simulink library "THBMemory"  (R2018b)
settings: Solver=ode45  StartTime=0.0  StopTime=10.0  RelTol=1e-3  EnableMultiTasking=on
settings Model: Creator=lena.frank  LastModifiedBy=P41573
settings DataIOCC: LimitDataPoints=on  SaveFormat=Array  SignalLoggingSaveFormat=ModelDataLogs
settings OptimizationCC: ExpressionDepthLimit=2147483647  LifeSpan=inf
settings DebuggingCC: UnderspecifiedInitializationDetection=Classic  MergeDetectMultiDrivingBlocksExec=none  SolverPrmCheckMsg=warning  FcnCallInpInsideContextMsg=warning  StateNameClashWarn=warning  SFUnexpectedBacktrackingDiag=warning  SFNoUnconditionalDefaultTransitionDiag=warning  SFExecutionAtInitializationDiag=none
settings HardwareCC: ProdBitPerPointer=32  ProdBitPerSizeT=32  ProdBitPerPtrDiffT=32  ProdLargestAtomicFloat=None  ProdIntDivRoundTo=Undefined  ProdEndianess=Unspecified  ProdWordSize=32  ProdHWDeviceType=32-bit Generic
settings ModelReferenceCC: PropagateSignalLabelsOutOfModel=off
settings SFSimCC: SimUseLocalCustomCode=off
settings RTWCC: RTWUseLocalCustomCode=off
settings CodeAppCC: StateflowObjectComments=on
settings GRTTargetCC: TargetLangStandard=C89/C90 (ANSI)  GeneratePreprocessorConditionals=Disable all  CombineOutputUpdateFcns=off  GRTInterface=on
settings ConfigComp: CovMetricSettings=dw  CovHtmlReporting=on  CovSaveCumulativeToWorkspaceVar=on  CovSaveSingleToWorkspaceVar=on  CovExternalEMLEnable=off

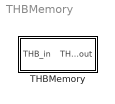
== system THBMemory ==
  THBMemory : Subsystem  InitFcn=load('THB.mat');  mask(THB Memory){ID=20001, T=20, mdot=0, p=1e5, FluidType=1, FluidMix=0, d=0.01, c=0, l=0, q=0, LH=1000, H=0, Annotation_ID=off, Annotation_T=off, Annotation_mdot=off, Annotation_p=off, Annotation_FluidType=off, Annotation_FluidMix=off, Annotation_d=off, Annotation_c=off, Annotation_l=off, Annotation_q=off, Annotation_LH=off, Annotation_H=off}
      mask prompts: ID "Fluid ID [1]"; T "Temperature [°C]"; mdot "Mass flow rate [kg/s]"; p "Pressure [Pa]"; FluidType "Fluid type [enum]"; FluidMix "Fluid mix [1]"; d "Diameter of the last piece [m]"; c "Constant pressure drop coefficient [Pa]"; l "Linear pressure drop coefficient [Pa/(kg/s)]"; q "Quadratic pressure drop coefficient [Pa/(kg/s)²]"; LH "Hydraulic inductance [1/m]"; H "Geodetic height [m]"; Annotation_ID "Fluid ID as annotation"; Annotation_T "Temperature as annoation"; Annotation_mdot "Mass flow rate as annoation"; Annotation_p "Pressure as annotation"; Annotation_FluidType "Fluid type as annotation"; Annotation_FluidMix "Fluid mix as annotation"; Annotation_d "Diameter of the last piece as annotation"; Annotation_c "Constant pressure drop coefficient as annotation"; Annotation_l "Linear pressure drop coefficient as annotation"; Annotation_q "Quadratic pressure drop coefficient as annotation"; Annotation_LH "Hydraulic inductance as annotation"; Annotation_H "Geodetic height as annotation"
      mask help: This is a memory block for a complete THB.
      mask init:
      | %annotations    
      | MaskValues=get_param(gcb,'MaskValues');
      | AnnotationString='';
      | if strcmp(MaskValues{13},'on') %ID
      |     if ~isempty(AnnotationString)
      |         AnnotationString=[AnnotationString,sprintf('\n')];
      |     end
      |     AnnotationString=[AnnotationString,'ID ',MaskValues{1}];
      | end
      |     
      | if strcmp(MaskValues{14},'on') %T
      |     if ~isempty(AnnotationString)
      |         AnnotationString=[AnnotationString,sprintf('\n')];
      |     end
      |     AnnotationString=[AnnotationString,MaskValues{2}, ' °C temperature'];
      | end
      |     
      | if strcmp(MaskValues{15},'on') %T
      |     if ~isempty(AnnotationString)
      |         AnnotationString=[AnnotationString,sprintf('\n')];
      |     end
      |     AnnotationString=[AnnotationString,MaskValues{3}, ' kg/s mass flow rate'];
      | end
      |     
      | if strcmp(MaskValues{16},'on') %p
      |     if ~isempty(AnnotationString)
      |         AnnotationString=[AnnotationString,sprintf('\n')];
      |     end
      |     AnnotationString=[AnnotationString,MaskValues{4}, ' Pa pressure'];
      | end
      | 
      | if strcmp(MaskValues{17},'on') %type
      |     if ~isempty(AnnotationString)
      |         AnnotationString=[AnnotationString,sprintf('\n')];
      |     end
      |     AnnotationString=[AnnotationString,'fluid type ',MaskValues{5}];
      | end
      |     
      | if strcmp(MaskValues{18},'on') %mix
      |     if ~isempty(AnnotationString)
      |         AnnotationString=[AnnotationString,sprintf('\n')];
      |     end
      |     AnnotationString=[AnnotationString,MaskValues{6}, ' fluid mix'];
      | end
      |     
      | if strcmp(MaskValues{19},'on') %d
      |     if ~isempty(AnnotationString)
      |         AnnotationString=[AnnotationString,sprintf('\n')];
      |     end
      |     AnnotationString=[AnnotationString,MaskValues{7}, ' m diameter last piece'];
      | end
      |     
      | if strcmp(MaskValues{20},'on') %c
      |     if ~isempty(AnnotationString)
      |         AnnotationString=[AnnotationString,sprintf('\n')];
      |     end
      |     AnnotationString=[AnnotationString,MaskValues{8}, ' Pa constant pressure loss coefficient'];
      | end
      |     
      | if strcmp(MaskValues{21},'on') %l
      |     if ~isempty(AnnotationString)
      |         AnnotationString=[AnnotationString,sprintf('\n')];
      |     end
      |     AnnotationString=[AnnotationString,MaskValues{9}, ' Pa/(kg/s) linear pressure loss coefficient'];
      | end
      |     
      | if strcmp(MaskValues{22},'on') %q
      |     if ~isempty(AnnotationString)
      |         AnnotationString=[AnnotationString,sprintf('\n')];
      |     end
      |     AnnotationString=[AnnotationString,MaskValues{10}, ' Pa/(kg/s)² quadratic pressure loss coefficient'];
      | end
      |     
      | if strcmp(MaskValues{23},'on') %LH
      |     if ~isempty(AnnotationString)
      |         AnnotationString=[AnnotationString,sprintf('\n')];
      |     end
      |     AnnotationString=[AnnotationString,MaskValues{11}, ' 1/m hydraulic inductance'];
      | end
      |     
      | if strcmp(MaskValues{24},'on') %H
      |     if ~isempty(AnnotationString)
      |         AnnotationString=[AnnotationString,sprintf('\n')];
      |     end
      |     AnnotationString=[AnnotationString,MaskValues{12}, ' m geodetic height'];
      | end
      |     
      | set_param(gcb,'AttributesFormatString',AnnotationString);
      | 
      | clear MaskValues AnnotationString;
      mask Help: web(fullfile(path_carnot('help'),'THBMemory.html'),'-helpbrowser')
      mask DialogControl ParameterTabVar0 Prompt: values
      mask DialogControl ParameterTabVar01 Prompt: annotations

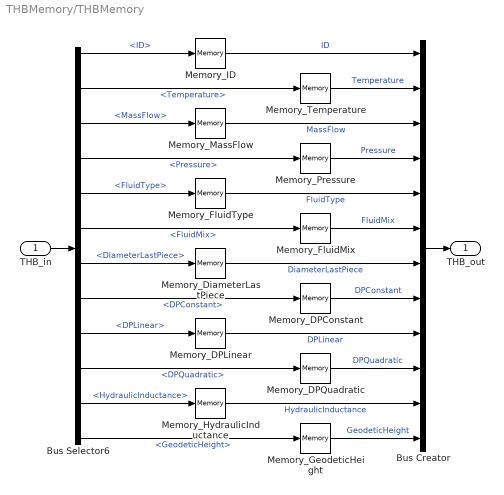
== system THBMemory/THBMemory ==
  THB_in : Inport  OutDataTypeStr=Bus: THB
  Bus Creator : BusCreator  Inputs=12
  Bus Selector6 : BusSelector  OutputSignals=ID,Temperature,MassFlow,Pressure,FluidType,FluidMix,DiameterLastPiece,DPConstant,DPLinear,DPQuadratic,HydraulicInductance,GeodeticHeight
  Memory_DPConstant : Memory  InitialCondition=c
  Memory_DPLinear : Memory  InitialCondition=l
  Memory_DPQuadratic : Memory  InitialCondition=q
  Memory_DiameterLastPiece : Memory  InitialCondition=d
  Memory_FluidMix : Memory  InitialCondition=FluidMix
  Memory_FluidType : Memory  InitialCondition=FluidType
  Memory_GeodeticHeight : Memory  InitialCondition=H
  Memory_HydraulicInductance : Memory  InitialCondition=LH
  Memory_ID : Memory  InitialCondition=ID
  Memory_MassFlow : Memory  InitialCondition=mdot
  Memory_Pressure : Memory  InitialCondition=p
  Memory_Temperature : Memory  InitialCondition=T
  THB_out : Outport
  wires:
  THB_in/1 -> Bus Selector6/1
  Bus Creator/1 -> THB_out/1
  Memory_HydraulicInductance/1 -> Bus Creator/11  "HydraulicInductance"
  Bus Selector6/11 -> Memory_HydraulicInductance/1  "<HydraulicInductance>"
  Memory_DPQuadratic/1 -> Bus Creator/10  "DPQuadratic"
  Bus Selector6/10 -> Memory_DPQuadratic/1  "<DPQuadratic>"
  Memory_DPLinear/1 -> Bus Creator/9  "DPLinear"
  Bus Selector6/9 -> Memory_DPLinear/1  "<DPLinear>"
  Memory_DPConstant/1 -> Bus Creator/8  "DPConstant"
  Bus Selector6/8 -> Memory_DPConstant/1  "<DPConstant>"
  Memory_DiameterLastPiece/1 -> Bus Creator/7  "DiameterLastPiece"
  Bus Selector6/7 -> Memory_DiameterLastPiece/1  "<DiameterLastPiece>"
  Memory_FluidMix/1 -> Bus Creator/6  "FluidMix"
  Bus Selector6/6 -> Memory_FluidMix/1  "<FluidMix>"
  Memory_FluidType/1 -> Bus Creator/5  "FluidType"
  Bus Selector6/5 -> Memory_FluidType/1  "<FluidType>"
  Memory_Pressure/1 -> Bus Creator/4  "Pressure"
  Bus Selector6/4 -> Memory_Pressure/1  "<Pressure>"
  Memory_MassFlow/1 -> Bus Creator/3  "MassFlow"
  Bus Selector6/3 -> Memory_MassFlow/1  "<MassFlow>"
  Memory_Temperature/1 -> Bus Creator/2  "Temperature"
  Bus Selector6/2 -> Memory_Temperature/1  "<Temperature>"
  Memory_ID/1 -> Bus Creator/1  "ID"
  Bus Selector6/1 -> Memory_ID/1  "<ID>"
  Memory_GeodeticHeight/1 -> Bus Creator/12  "GeodeticHeight"
  Bus Selector6/12 -> Memory_GeodeticHeight/1  "<GeodeticHeight>"
